simulink model "Controlador_de_corriente_estimador"  (R2014b)
settings: Solver=ode23t  StartTime=0.0  StopTime=15e-3  RelTol=1e-3
model workspace (MAT data in the model file):
  kh = Simulink.Parameter
  kh.Value = 0.0533333333333
  kh.DataType = 'auto'
  C1 = Simulink.Parameter
  C1.Value = 1e-06
  C1.DataType = 'auto'
  R1 = Simulink.Parameter
  R1.Value = 25000
  R1.DataType = 'auto'
  RL = Simulink.Parameter
  RL.Value = 0.2
  RL.DataType = 'auto'
  Lyo = Simulink.Parameter
  Lyo.Value = 0.08
  Lyo.DataType = 'auto'
values from neighbouring files (symbols this model uses):
  R1 = 25e3    (= 25000)    [compensacion_derivador_con_mcp660.m]
settings Model: Creator=Javi  LastModifiedBy=Javi

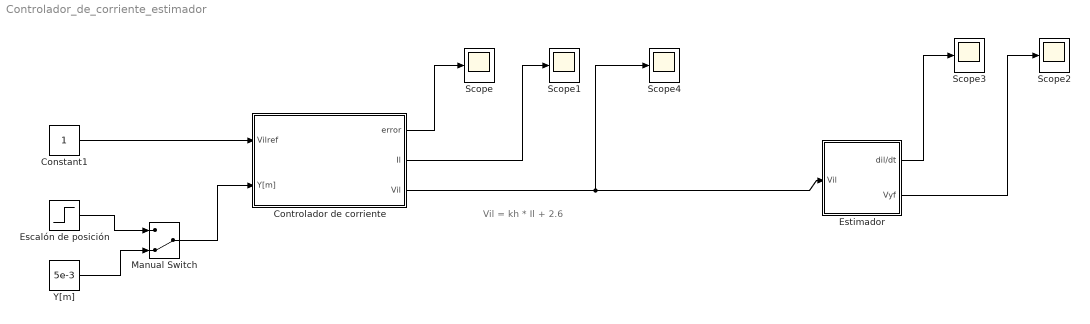
== system Controlador_de_corriente_estimador ==
  note: Vil = kh * Il + 2.6
  Constant1 : Constant
  "Controlador de corriente " : Subsystem
  "Escalón de posición " : Step  Time=10e-3  Before=2e-3  After=5e-3  SampleTime=0
  "Estimador " : Subsystem
  Manual Switch : ManualSwitch  CurrentSetting=0
  Scope{,1..4} (5 alike) : Scope
      Scope settings: TimeRange=0.015  YMin=2.4  YMax=3.1
      Scope1 settings: TimeRange=0.015  YMin=0  YMax=14
      Scope2 settings: TimeRange=0.015  YMin=3  YMax=6  SaveName=ScopeData2
      Scope3 settings: TimeRange=0.015  YMin=0.5  YMax=4.5  SaveName=ScopeData3
      Scope4 settings: TimeRange=0.015  YMin=2.5  YMax=3.2  SaveName=ScopeData4
  Y[m] : Constant  Value=5e-3
  wires:
  "Controlador de corriente "/1("error ") -> Scope/1
  "Controlador de corriente "/2("Il ") -> Scope1/1
  "Estimador "/1(dil/dt) -> Scope3/1
  "Estimador "/2(Vyf) -> Scope2/1
  "Controlador de corriente "/3("Vil ") -> Scope4/1, "Estimador "/1(Vil)
  Constant1/1 -> "Controlador de corriente "/1("Vilref ")
  Y[m]/1 -> Manual Switch/2
  "Escalón de posición "/1 -> Manual Switch/1
  Manual Switch/1 -> "Controlador de corriente "/2("Y[m] ")

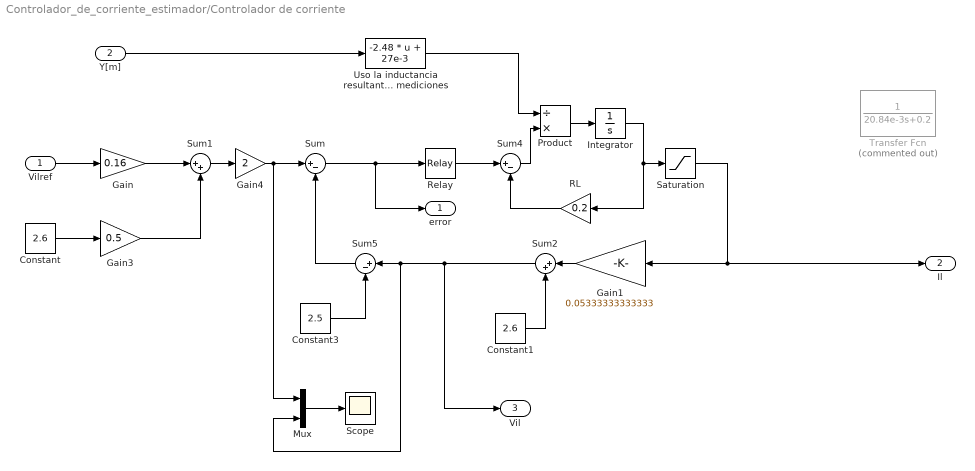
== system Controlador_de_corriente_estimador/Controlador de corriente  ==
  "Vilref " : Inport
  "Y[m] " : Inport  Port=2
  Constant : Constant  Value=2.6
  Constant1 : Constant  Value=2.6
  Constant3 : Constant  Value=2.5
  Gain : Gain  Gain=0.16
  Gain1 : Gain  Gain=0.05333333333333
  Gain3 : Gain  Gain=0.5
  Gain4 : Gain  Gain=2
  Integrator : Integrator
  Mux : Mux  Inputs=2
  Product : Product  Inputs=/*
  RL : Gain  Gain=0.2
  Relay : Relay  OnSwitchValue=2.5125  OffSwitchValue=2.4875  OnOutputValue=24  OffOutputValue=-24
  Saturation : Saturate  UpperLimit=40  LowerLimit=0
  Scope : Scope
      settings: SaveName=ScopeData2
  Sum : Sum  Inputs=|+-
  Sum1 : Sum  Inputs=|++
  Sum2 : Sum  Inputs=|++
  Sum4 : Sum  Inputs=|+-
  Sum5 : Sum  Inputs=|+-
  Transfer Fcn : TransferFcn  Commented=on  Denominator=[20.84e-3 0.2]
  "Uso la inductancia resultante de las mediciones " : Fcn  Expr=-2.48 * u + 27e-3
  "error " : Outport
  "Il " : Outport  Port=2
  "Vil " : Outport  Port=3
  wires:
  Sum1/1 -> Gain4/1
  Gain4/1 -> Sum/1, Mux/1
  Gain3/1 -> Sum1/2
  Gain/1 -> Sum1/1
  Saturation/1 -> "Il "/1, Gain1/1
  Constant/1 -> Gain3/1
  "Vilref "/1 -> Gain/1
  Mux/1 -> Scope/1
  Constant1/1 -> Sum2/2
  Gain1/1 -> Sum2/1
  Sum2/1 -> "Vil "/1, Sum5/1, Mux/2
  Sum/1 -> Relay/1, "error "/1
  Relay/1 -> Sum4/1
  Integrator/1 -> RL/1, Saturation/1
  Product/1 -> Integrator/1
  Sum4/1 -> Product/2
  "Y[m] "/1 -> "Uso la inductancia resultante de las mediciones "/1
  "Uso la inductancia resultante de las mediciones "/1 -> Product/1
  Sum5/1 -> Sum/2
  Constant3/1 -> Sum5/2
  RL/1 -> Sum4/2

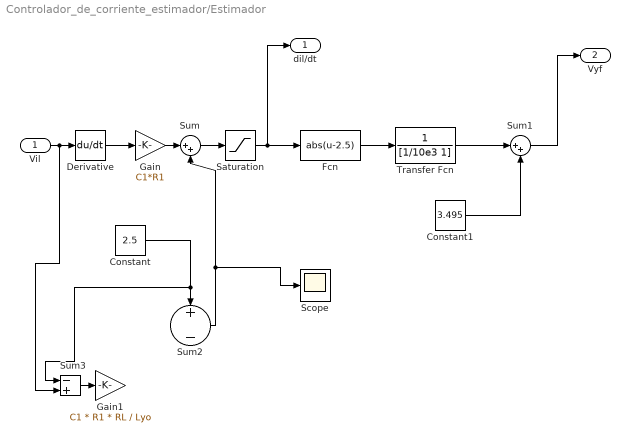
== system Controlador_de_corriente_estimador/Estimador  ==
  Vil : Inport
  Constant : Constant  Value=2.5
  Constant1 : Constant  Value=3.495
  Derivative : Derivative  CoefficientInTFapproximation=10*1e-6
  Fcn : Fcn  Expr=abs(u-2.5)
  Gain : Gain  Gain=C1*R1
  Gain1 : Gain  Gain=C1 * R1 * RL / Lyo
  Saturation : Saturate  UpperLimit=5  LowerLimit=0
  Scope : Scope
      settings: SaveName=ScopeData5
  Sum : Sum  Inputs=|++
  Sum1 : Sum  Inputs=|++
  Sum2 : Sum  Inputs=+-
  Sum3 : Sum  Inputs=-+
  Transfer Fcn : TransferFcn  Denominator=[1/10e3 1]
  dil/dt : Outport
  Vyf : Outport  Port=2
  wires:
  Vil/1 -> Sum3/2, Derivative/1
  Derivative/1 -> Gain/1
  Saturation/1 -> Fcn/1, dil/dt/1
  Sum/1 -> Saturation/1
  Constant/1 -> Sum3/1, Sum2/1
  Fcn/1 -> Transfer Fcn/1
  Sum1/1 -> Vyf/1
  Transfer Fcn/1 -> Sum1/1
  Constant1/1 -> Sum1/2
  Sum2/1 -> Scope/1, Sum/2
  Sum3/1 -> Gain1/1
  Gain/1 -> Sum/1
